simulink model "pil_top_am13x"  (R2025b)
settings: Solver=FixedStepAuto  StartTime=0.0  StopTime=1  RelTol=1e-3  EnableMultiTasking=on
libraries: simulink x1
settings Model: SILPILSystemUnderTest=refmodels  CodeVerificationMode=processor-in-the-loop (pil)  Creator=a1255762  LastModifiedBy=a1255762
settings OptimizationCC: DefaultUnderspecifiedDataType=single  EnhancedBackFolding=on  PassReuseOutputArgsThreshold=0.0  MaxStackSize=64  OptimizeBlockOrder=speed  DifferentSizesBufferReuse=on  OptimizationCustomize=off
settings DebuggingCC: ParameterPrecisionLossMsg=none  ParameterTunabilityLossMsg=error
settings SFSimCC: MATLABDynamicMemAlloc=off
settings RTWCC: GenerateReport=on  BuildConfiguration=Faster Runs  LaunchReport=on  CodeExecutionProfiling=on
settings CodeAppCC: ForceParamTrailComments=on  MaxIdLength=256.0  OperatorAnnotations=on
settings GRTTargetCC: TargetLangStandard=C89/C90 (ANSI)

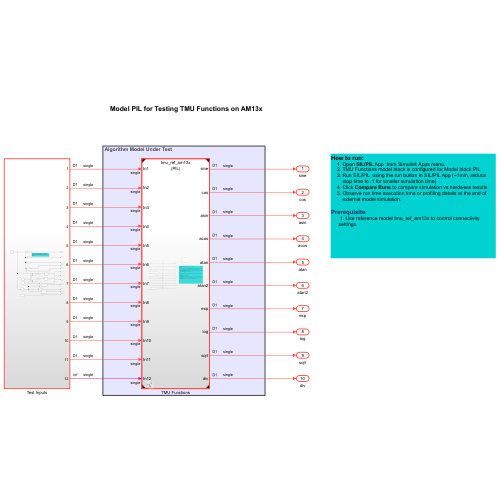
[thumbnail: Simulink's stored preview of the top-level diagram]
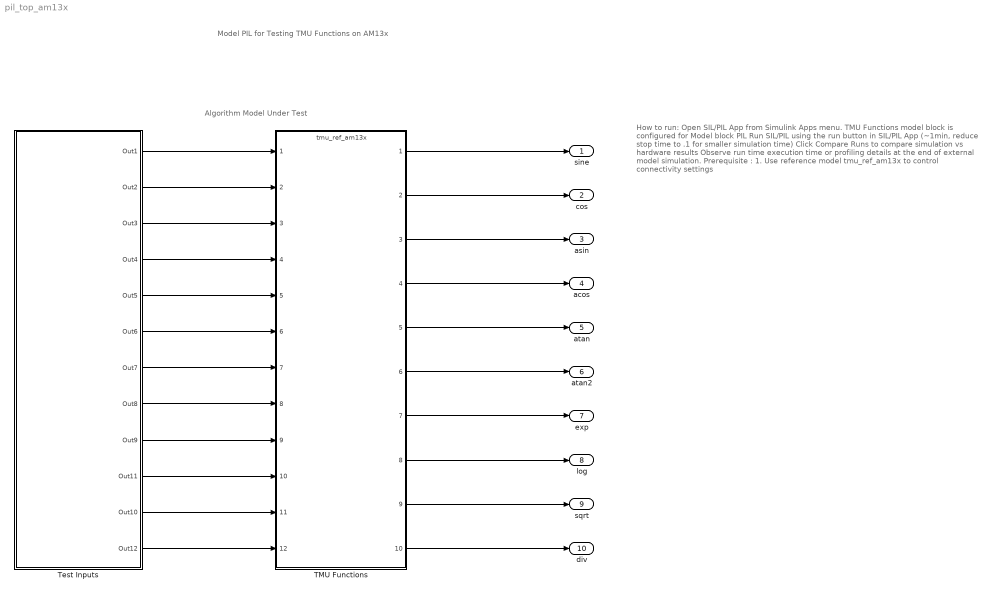
== system pil_top_am13x ==
  note: How to run:
      | Open SIL/PIL App from Simulink Apps menu.
      | TMU Functions model block is configured for Model block PIL
      | Run SIL/PIL using the run button in SIL/PIL App (~1min, reduce stop time to .1 for smaller simulation time)
      | Click Compare Runs to compare simulation vs hardware results
      | Observe run time execution time or profiling details at the end of external model simulation.
      |
      | Prerequisite :
      | 1. Use reference model tmu_ref_am13x to control connectivity settings
  note: Model PIL for Testing TMU Functions on AM13x
  note: Algorithm Model Under Test
  TMU Functions : ModelReference  ModelNameDialog=tmu_ref_am13x.slx  SimulationMode=Processor-in-the-loop (PIL)  ModelReferenceVersion=1.124
  Test Inputs : Subsystem
  sine : Outport
  cos : Outport  Port=2
  asin : Outport  Port=3
  acos : Outport  Port=4
  atan : Outport  Port=5
  atan2 : Outport  Port=6
  exp : Outport  Port=7
  log : Outport  Port=8
  sqrt : Outport  Port=9
  div : Outport  Port=10
  wires:
  Test Inputs/1(Out1) -> TMU Functions/1
  Test Inputs/2(Out2) -> TMU Functions/2
  Test Inputs/3(Out3) -> TMU Functions/3
  Test Inputs/4(Out4) -> TMU Functions/4
  Test Inputs/5(Out5) -> TMU Functions/5
  Test Inputs/6(Out6) -> TMU Functions/6
  Test Inputs/7(Out7) -> TMU Functions/7
  Test Inputs/8(Out8) -> TMU Functions/8
  Test Inputs/9(Out9) -> TMU Functions/9
  Test Inputs/10(Out11) -> TMU Functions/10
  Test Inputs/11(Out10) -> TMU Functions/11
  Test Inputs/12(Out12) -> TMU Functions/12
  TMU Functions/1 -> sine/1
  TMU Functions/2 -> cos/1
  TMU Functions/3 -> asin/1
  TMU Functions/4 -> acos/1
  TMU Functions/5 -> atan/1
  TMU Functions/6 -> atan2/1
  TMU Functions/7 -> exp/1
  TMU Functions/8 -> log/1
  TMU Functions/9 -> sqrt/1
  TMU Functions/10 -> div/1

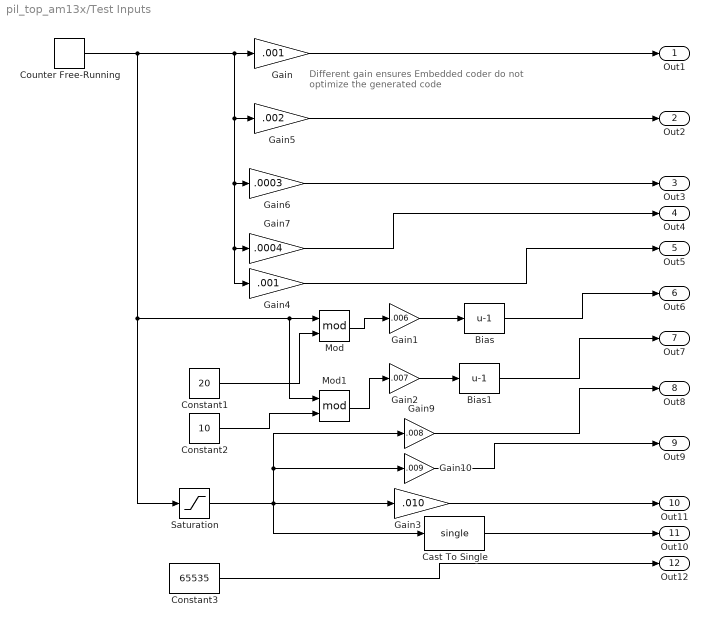
== system pil_top_am13x/Test Inputs ==
  note: Different gain ensures Embedded coder do not optimize the generated code
  Bias : Bias  Bias=-1  SaturateOnIntegerOverflow=off
  Bias1 : Bias  Bias=-1  SaturateOnIntegerOverflow=off
  Cast To Single : DataTypeConversion  OutDataTypeStr=single  SaturateOnIntegerOverflow=off  RndMeth=Floor
  Constant1 : Constant  Value=20  OutDataTypeStr=uint16
  Constant2 : Constant  Value=10  OutDataTypeStr=uint16
  Constant3 : Constant  Value=65535  OutDataTypeStr=single
  Counter Free-Running : simulink/Sources/Counter Free-Running  NumBits=16  tsamp=.001
  Gain : Gain  Gain=.001  OutDataTypeStr=single
  Gain1 : Gain  Gain=.006  OutDataTypeStr=single
  Gain10 : Gain  Gain=.009  OutDataTypeStr=single
  Gain2 : Gain  Gain=.007  OutDataTypeStr=single
  Gain3 : Gain  Gain=.010  OutDataTypeStr=single
  Gain4 : Gain  Gain=.001  OutDataTypeStr=single
  Gain5 : Gain  Gain=.002  OutDataTypeStr=single
  Gain6 : Gain  Gain=.0003  OutDataTypeStr=single
  Gain7 : Gain  Gain=.0004  OutDataTypeStr=single
  Gain9 : Gain  Gain=.008  OutDataTypeStr=single
  Mod : Math  Operator=mod
  Mod1 : Math  Operator=mod
  Saturation : Saturate  UpperLimit=65535  LowerLimit=1
  Out1 : Outport
  Out2 : Outport  Port=2
  Out3 : Outport  Port=3
  Out4 : Outport  Port=4
  Out5 : Outport  Port=5
  Out6 : Outport  Port=6
  Out7 : Outport  Port=7
  Out8 : Outport  Port=8
  Out9 : Outport  Port=9
  Out11 : Outport  Port=10
  Out10 : Outport  Port=11
  Out12 : Outport  Port=12
  wires:
  Bias1/1 -> Out7/1
  Counter Free-Running/1 -> Saturation/1, Mod/1, Mod1/1, Gain4/1, Gain7/1, Gain6/1, Gain5/1, Gain/1
  Saturation/1 -> Gain10/1, Gain9/1, Cast To Single/1, Gain3/1
  Gain9/1 -> Out8/1
  Constant3/1 -> Out12/1
  Mod1/1 -> Gain2/1
  Gain1/1 -> Bias/1
  Gain3/1 -> Out11/1
  Mod/1 -> Gain1/1
  Constant2/1 -> Mod1/2
  Gain10/1 -> Out9/1
  Gain2/1 -> Bias1/1
  Gain5/1 -> Out2/1
  Gain6/1 -> Out3/1
  Constant1/1 -> Mod/2
  Gain7/1 -> Out4/1
  Bias/1 -> Out6/1
  Gain/1 -> Out1/1
  Gain4/1 -> Out5/1
  Cast To Single/1 -> Out10/1
